simulink model "model_cnn"  (R2020a)
settings: Solver=VariableStepAuto  StartTime=0.0  StopTime=1e6/fs  RelTol=1e-3
PreLoadFcn:
  | setup_imports;
  | %dense2_numerictype = fixdt(1,18,10);
  | %conv1_numerictype = fixdt(1,18,21);
InitFcn:
  | % Intermediate signal dimensions
  | input_dim = [1, 2, 128];
  | layer1_dim = hInterConvLayerDims([1,3,1,64],input_dim,1); % dims : [C,H,W]
  | layer2_dim = hInterConvLayerDims([2,3,64,16],layer1_dim,1);% dims : [C,H,W]
  | layer3_dim = [1,128];
  | 
  | % Conv Layer 1 dimensions
  | conv1_dims = struct(...
  |     'input_dim',    input_dim,...       input_dim = C,H,W
  |     'filter_dim',   [1, 3, 1, 64],...  filter_dim = K,J,C,N
  |     'stride',       1,...
  |     'row_output',   3,...
  |     'output_dim',   layer1_dim);
  | 
  | % Conv Layer 2 dimensions
  | conv2_dims = struct(...
  |     'input_dim',    layer1_dim,...      input = C,H.W
  |     'filter_dim',   [2, 3, 64, 16],...  filter_dim = K,J,C,N
  |     'stride',       1,...
  |     'row_output',   2*3*64,...
  |     'output_dim',   layer2_dim);
  | 
  | % Dense Layer 1 dimensions
  | dense1_dims = struct(...
  |     'input_dim',    layer2_dim,...      input = C,H,W
  |     'weight_dim',   [1984, 128],...     weight_dim = H,W
  |     'output_dim',   layer3_dim);
  | 
  | % Load saved weights and input
  | setup_imports;
  | 
  | fs = 128e6;
  | fs_axi = 100e6;
  | R = 32;
values from neighbouring files (symbols this model uses):
  datatypeInput = X_test.numerictype    [setup_imports.m]
  gemm_wconv1 = fi(hInterleaveFilters(Wconv1),1,16)    [setup_imports.m]
  gemm_wconv2 = fi(hInterleaveFilters(Wconv2),1,16)    [setup_imports.m]
  wdense1 = fi(Wdense1,1,16)    [setup_imports.m]
  wdense2 = fi(Wdense2,1,16)    [setup_imports.m]
undefined symbols (not defined in the file or in its folder): ltehdlRAMinitPO2
libraries: hdlsllib x1022, dspsigops x3, dspsrcs4 x2
(part 5 of 23)

== system model_cnn/HDL CNN Model/Conv Layer 1/Layer 1 Mat-Vec Multiplier/adder54 ==
  In1 : Inport
  In2 : Inport  Port=2
  In3 : Inport  Port=3
  Data Type Conversion : DataTypeConversion  OutDataTypeStr=conv1_numerictype
  Multiply-Accumulate : hdlsllib/HDL Operations/Multiply-Accumulate  opMode=Streaming - using Number of Samples  initValueSetting=Dialog  initValue=0  initValueSetting2=Dialog  initValue2=0  initValueSetting3=Dialog  initValue3=0  num_samples=3  RndMeth2=Floor  RndMeth3=Floor  datatype2=Inherit: Inherit via back propagation  datatype3=accumoutdatatype1  validOut=on  endInandOut=on  startOut=on  countOut=on  dim=-1  DoSatur=off  parallel=off
      settings: SourceProductBaseCode=SL
  Terminator : Terminator
  Terminator1 : Terminator
  Terminator2 : Terminator
  dataOut : Outport
  wires:
  Data Type Conversion/1 -> dataOut/1
  ? -> Terminator1/1  "validOut"
  In2/1 -> Multiply-Accumulate/1
  In3/1 -> ?
  Multiply-Accumulate/1 -> Data Type Conversion/1
  ? -> Terminator/1  "countOut"
  In1/1 -> Multiply-Accumulate/2
  ? -> Terminator2/1  "vectorOutValid"

== system model_cnn/HDL CNN Model/Conv Layer 1/Layer 1 Mat-Vec Multiplier/adder55 ==
  In1 : Inport
  In2 : Inport  Port=2
  In3 : Inport  Port=3
  Data Type Conversion : DataTypeConversion  OutDataTypeStr=conv1_numerictype
  Multiply-Accumulate : hdlsllib/HDL Operations/Multiply-Accumulate  opMode=Streaming - using Number of Samples  initValueSetting=Dialog  initValue=0  initValueSetting2=Dialog  initValue2=0  initValueSetting3=Dialog  initValue3=0  num_samples=3  RndMeth2=Floor  RndMeth3=Floor  datatype2=Inherit: Inherit via back propagation  datatype3=accumoutdatatype1  validOut=on  endInandOut=on  startOut=on  countOut=on  dim=-1  DoSatur=off  parallel=off
      settings: SourceProductBaseCode=SL
  Terminator : Terminator
  Terminator1 : Terminator
  Terminator2 : Terminator
  dataOut : Outport
  wires:
  Data Type Conversion/1 -> dataOut/1
  ? -> Terminator1/1  "validOut"
  In2/1 -> Multiply-Accumulate/1
  In3/1 -> ?
  Multiply-Accumulate/1 -> Data Type Conversion/1
  ? -> Terminator/1  "countOut"
  In1/1 -> Multiply-Accumulate/2
  ? -> Terminator2/1  "vectorOutValid"

== system model_cnn/HDL CNN Model/Conv Layer 1/Layer 1 Mat-Vec Multiplier/adder56 ==
  In1 : Inport
  In2 : Inport  Port=2
  In3 : Inport  Port=3
  Data Type Conversion : DataTypeConversion  OutDataTypeStr=conv1_numerictype
  Multiply-Accumulate : hdlsllib/HDL Operations/Multiply-Accumulate  opMode=Streaming - using Number of Samples  initValueSetting=Dialog  initValue=0  initValueSetting2=Dialog  initValue2=0  initValueSetting3=Dialog  initValue3=0  num_samples=3  RndMeth2=Floor  RndMeth3=Floor  datatype2=Inherit: Inherit via back propagation  datatype3=accumoutdatatype1  validOut=on  endInandOut=on  startOut=on  countOut=on  dim=-1  DoSatur=off  parallel=off
      settings: SourceProductBaseCode=SL
  Terminator : Terminator
  Terminator1 : Terminator
  Terminator2 : Terminator
  dataOut : Outport
  wires:
  Data Type Conversion/1 -> dataOut/1
  ? -> Terminator1/1  "validOut"
  In2/1 -> Multiply-Accumulate/1
  In3/1 -> ?
  Multiply-Accumulate/1 -> Data Type Conversion/1
  ? -> Terminator/1  "countOut"
  In1/1 -> Multiply-Accumulate/2
  ? -> Terminator2/1  "vectorOutValid"

== system model_cnn/HDL CNN Model/Conv Layer 1/Layer 1 Mat-Vec Multiplier/adder57 ==
  In1 : Inport
  In2 : Inport  Port=2
  In3 : Inport  Port=3
  Data Type Conversion : DataTypeConversion  OutDataTypeStr=conv1_numerictype
  Multiply-Accumulate : hdlsllib/HDL Operations/Multiply-Accumulate  opMode=Streaming - using Number of Samples  initValueSetting=Dialog  initValue=0  initValueSetting2=Dialog  initValue2=0  initValueSetting3=Dialog  initValue3=0  num_samples=3  RndMeth2=Floor  RndMeth3=Floor  datatype2=Inherit: Inherit via back propagation  datatype3=accumoutdatatype1  validOut=on  endInandOut=on  startOut=on  countOut=on  dim=-1  DoSatur=off  parallel=off
      settings: SourceProductBaseCode=SL
  Terminator : Terminator
  Terminator1 : Terminator
  Terminator2 : Terminator
  dataOut : Outport
  wires:
  Data Type Conversion/1 -> dataOut/1
  ? -> Terminator1/1  "validOut"
  In2/1 -> Multiply-Accumulate/1
  In3/1 -> ?
  Multiply-Accumulate/1 -> Data Type Conversion/1
  ? -> Terminator/1  "countOut"
  In1/1 -> Multiply-Accumulate/2
  ? -> Terminator2/1  "vectorOutValid"

== system model_cnn/HDL CNN Model/Conv Layer 1/Layer 1 Mat-Vec Multiplier/adder58 ==
  In1 : Inport
  In2 : Inport  Port=2
  In3 : Inport  Port=3
  Data Type Conversion : DataTypeConversion  OutDataTypeStr=conv1_numerictype
  Multiply-Accumulate : hdlsllib/HDL Operations/Multiply-Accumulate  opMode=Streaming - using Number of Samples  initValueSetting=Dialog  initValue=0  initValueSetting2=Dialog  initValue2=0  initValueSetting3=Dialog  initValue3=0  num_samples=3  RndMeth2=Floor  RndMeth3=Floor  datatype2=Inherit: Inherit via back propagation  datatype3=accumoutdatatype1  validOut=on  endInandOut=on  startOut=on  countOut=on  dim=-1  DoSatur=off  parallel=off
      settings: SourceProductBaseCode=SL
  Terminator : Terminator
  Terminator1 : Terminator
  Terminator2 : Terminator
  dataOut : Outport
  wires:
  Data Type Conversion/1 -> dataOut/1
  ? -> Terminator1/1  "validOut"
  In2/1 -> Multiply-Accumulate/1
  In3/1 -> ?
  Multiply-Accumulate/1 -> Data Type Conversion/1
  ? -> Terminator/1  "countOut"
  In1/1 -> Multiply-Accumulate/2
  ? -> Terminator2/1  "vectorOutValid"

== system model_cnn/HDL CNN Model/Conv Layer 1/Layer 1 Mat-Vec Multiplier/adder59 ==
  In1 : Inport
  In2 : Inport  Port=2
  In3 : Inport  Port=3
  Data Type Conversion : DataTypeConversion  OutDataTypeStr=conv1_numerictype
  Multiply-Accumulate : hdlsllib/HDL Operations/Multiply-Accumulate  opMode=Streaming - using Number of Samples  initValueSetting=Dialog  initValue=0  initValueSetting2=Dialog  initValue2=0  initValueSetting3=Dialog  initValue3=0  num_samples=3  RndMeth2=Floor  RndMeth3=Floor  datatype2=Inherit: Inherit via back propagation  datatype3=accumoutdatatype1  validOut=on  endInandOut=on  startOut=on  countOut=on  dim=-1  DoSatur=off  parallel=off
      settings: SourceProductBaseCode=SL
  Terminator : Terminator
  Terminator1 : Terminator
  Terminator2 : Terminator
  dataOut : Outport
  wires:
  Data Type Conversion/1 -> dataOut/1
  ? -> Terminator1/1  "validOut"
  In2/1 -> Multiply-Accumulate/1
  In3/1 -> ?
  Multiply-Accumulate/1 -> Data Type Conversion/1
  ? -> Terminator/1  "countOut"
  In1/1 -> Multiply-Accumulate/2
  ? -> Terminator2/1  "vectorOutValid"

== system model_cnn/HDL CNN Model/Conv Layer 1/Layer 1 Mat-Vec Multiplier/adder6 ==
  In1 : Inport
  In2 : Inport  Port=2
  In3 : Inport  Port=3
  Data Type Conversion : DataTypeConversion  OutDataTypeStr=conv1_numerictype
  Multiply-Accumulate : hdlsllib/HDL Operations/Multiply-Accumulate  opMode=Streaming - using Number of Samples  initValueSetting=Dialog  initValue=0  initValueSetting2=Dialog  initValue2=0  initValueSetting3=Dialog  initValue3=0  num_samples=3  RndMeth2=Floor  RndMeth3=Floor  datatype2=Inherit: Inherit via back propagation  datatype3=accumoutdatatype1  validOut=on  endInandOut=on  startOut=on  countOut=on  dim=-1  DoSatur=off  parallel=off
      settings: SourceProductBaseCode=SL
  Terminator : Terminator
  Terminator1 : Terminator
  Terminator2 : Terminator
  dataOut : Outport
  wires:
  Data Type Conversion/1 -> dataOut/1
  ? -> Terminator1/1  "validOut"
  In2/1 -> Multiply-Accumulate/1
  In3/1 -> ?
  Multiply-Accumulate/1 -> Data Type Conversion/1
  ? -> Terminator/1  "countOut"
  In1/1 -> Multiply-Accumulate/2
  ? -> Terminator2/1  "vectorOutValid"

== system model_cnn/HDL CNN Model/Conv Layer 1/Layer 1 Mat-Vec Multiplier/adder60 ==
  In1 : Inport
  In2 : Inport  Port=2
  In3 : Inport  Port=3
  Data Type Conversion : DataTypeConversion  OutDataTypeStr=conv1_numerictype
  Multiply-Accumulate : hdlsllib/HDL Operations/Multiply-Accumulate  opMode=Streaming - using Number of Samples  initValueSetting=Dialog  initValue=0  initValueSetting2=Dialog  initValue2=0  initValueSetting3=Dialog  initValue3=0  num_samples=3  RndMeth2=Floor  RndMeth3=Floor  datatype2=Inherit: Inherit via back propagation  datatype3=accumoutdatatype1  validOut=on  endInandOut=on  startOut=on  countOut=on  dim=-1  DoSatur=off  parallel=off
      settings: SourceProductBaseCode=SL
  Terminator : Terminator
  Terminator1 : Terminator
  Terminator2 : Terminator
  dataOut : Outport
  wires:
  Data Type Conversion/1 -> dataOut/1
  ? -> Terminator1/1  "validOut"
  In2/1 -> Multiply-Accumulate/1
  In3/1 -> ?
  Multiply-Accumulate/1 -> Data Type Conversion/1
  ? -> Terminator/1  "countOut"
  In1/1 -> Multiply-Accumulate/2
  ? -> Terminator2/1  "vectorOutValid"

== system model_cnn/HDL CNN Model/Conv Layer 1/Layer 1 Mat-Vec Multiplier/adder61 ==
  In1 : Inport
  In2 : Inport  Port=2
  In3 : Inport  Port=3
  Data Type Conversion : DataTypeConversion  OutDataTypeStr=conv1_numerictype
  Multiply-Accumulate : hdlsllib/HDL Operations/Multiply-Accumulate  opMode=Streaming - using Number of Samples  initValueSetting=Dialog  initValue=0  initValueSetting2=Dialog  initValue2=0  initValueSetting3=Dialog  initValue3=0  num_samples=3  RndMeth2=Floor  RndMeth3=Floor  datatype2=Inherit: Inherit via back propagation  datatype3=accumoutdatatype1  validOut=on  endInandOut=on  startOut=on  countOut=on  dim=-1  DoSatur=off  parallel=off
      settings: SourceProductBaseCode=SL
  Terminator : Terminator
  Terminator1 : Terminator
  Terminator2 : Terminator
  dataOut : Outport
  wires:
  Data Type Conversion/1 -> dataOut/1
  ? -> Terminator1/1  "validOut"
  In2/1 -> Multiply-Accumulate/1
  In3/1 -> ?
  Multiply-Accumulate/1 -> Data Type Conversion/1
  ? -> Terminator/1  "countOut"
  In1/1 -> Multiply-Accumulate/2
  ? -> Terminator2/1  "vectorOutValid"

== system model_cnn/HDL CNN Model/Conv Layer 1/Layer 1 Mat-Vec Multiplier/adder62 ==
  In1 : Inport
  In2 : Inport  Port=2
  In3 : Inport  Port=3
  Data Type Conversion : DataTypeConversion  OutDataTypeStr=conv1_numerictype
  Multiply-Accumulate : hdlsllib/HDL Operations/Multiply-Accumulate  opMode=Streaming - using Number of Samples  initValueSetting=Dialog  initValue=0  initValueSetting2=Dialog  initValue2=0  initValueSetting3=Dialog  initValue3=0  num_samples=3  RndMeth2=Floor  RndMeth3=Floor  datatype2=Inherit: Inherit via back propagation  datatype3=accumoutdatatype1  validOut=on  endInandOut=on  startOut=on  countOut=on  dim=-1  DoSatur=off  parallel=off
      settings: SourceProductBaseCode=SL
  Terminator : Terminator
  Terminator1 : Terminator
  Terminator2 : Terminator
  dataOut : Outport
  wires:
  Data Type Conversion/1 -> dataOut/1
  ? -> Terminator1/1  "validOut"
  In2/1 -> Multiply-Accumulate/1
  In3/1 -> ?
  Multiply-Accumulate/1 -> Data Type Conversion/1
  ? -> Terminator/1  "countOut"
  In1/1 -> Multiply-Accumulate/2
  ? -> Terminator2/1  "vectorOutValid"

== system model_cnn/HDL CNN Model/Conv Layer 1/Layer 1 Mat-Vec Multiplier/adder63 ==
  In1 : Inport
  In2 : Inport  Port=2
  In3 : Inport  Port=3
  Data Type Conversion : DataTypeConversion  OutDataTypeStr=conv1_numerictype
  Multiply-Accumulate : hdlsllib/HDL Operations/Multiply-Accumulate  opMode=Streaming - using Number of Samples  initValueSetting=Dialog  initValue=0  initValueSetting2=Dialog  initValue2=0  initValueSetting3=Dialog  initValue3=0  num_samples=3  RndMeth2=Floor  RndMeth3=Floor  datatype2=Inherit: Inherit via back propagation  datatype3=accumoutdatatype1  validOut=on  endInandOut=on  startOut=on  countOut=on  dim=-1  DoSatur=off  parallel=off
      settings: SourceProductBaseCode=SL
  Terminator : Terminator
  Terminator1 : Terminator
  Terminator2 : Terminator
  dataOut : Outport
  wires:
  Data Type Conversion/1 -> dataOut/1
  ? -> Terminator1/1  "validOut"
  In2/1 -> Multiply-Accumulate/1
  In3/1 -> ?
  Multiply-Accumulate/1 -> Data Type Conversion/1
  ? -> Terminator/1  "countOut"
  In1/1 -> Multiply-Accumulate/2
  ? -> Terminator2/1  "vectorOutValid"

== system model_cnn/HDL CNN Model/Conv Layer 1/Layer 1 Mat-Vec Multiplier/adder7 ==
  In1 : Inport
  In2 : Inport  Port=2
  In3 : Inport  Port=3
  Data Type Conversion : DataTypeConversion  OutDataTypeStr=conv1_numerictype
  Multiply-Accumulate : hdlsllib/HDL Operations/Multiply-Accumulate  opMode=Streaming - using Number of Samples  initValueSetting=Dialog  initValue=0  initValueSetting2=Dialog  initValue2=0  initValueSetting3=Dialog  initValue3=0  num_samples=3  RndMeth2=Floor  RndMeth3=Floor  datatype2=Inherit: Inherit via back propagation  datatype3=accumoutdatatype1  validOut=on  endInandOut=on  startOut=on  countOut=on  dim=-1  DoSatur=off  parallel=off
      settings: SourceProductBaseCode=SL
  Terminator : Terminator
  Terminator1 : Terminator
  Terminator2 : Terminator
  dataOut : Outport
  wires:
  Data Type Conversion/1 -> dataOut/1
  ? -> Terminator1/1  "validOut"
  In2/1 -> Multiply-Accumulate/1
  In3/1 -> ?
  Multiply-Accumulate/1 -> Data Type Conversion/1
  ? -> Terminator/1  "countOut"
  In1/1 -> Multiply-Accumulate/2
  ? -> Terminator2/1  "vectorOutValid"

== system model_cnn/HDL CNN Model/Conv Layer 1/Layer 1 Mat-Vec Multiplier/adder8 ==
  In1 : Inport
  In2 : Inport  Port=2
  In3 : Inport  Port=3
  Data Type Conversion : DataTypeConversion  OutDataTypeStr=conv1_numerictype
  Multiply-Accumulate : hdlsllib/HDL Operations/Multiply-Accumulate  opMode=Streaming - using Number of Samples  initValueSetting=Dialog  initValue=0  initValueSetting2=Dialog  initValue2=0  initValueSetting3=Dialog  initValue3=0  num_samples=3  RndMeth2=Floor  RndMeth3=Floor  datatype2=Inherit: Inherit via back propagation  datatype3=accumoutdatatype1  validOut=on  endInandOut=on  startOut=on  countOut=on  dim=-1  DoSatur=off  parallel=off
      settings: SourceProductBaseCode=SL
  Terminator : Terminator
  Terminator1 : Terminator
  Terminator2 : Terminator
  dataOut : Outport
  wires:
  Data Type Conversion/1 -> dataOut/1
  ? -> Terminator1/1  "validOut"
  In2/1 -> Multiply-Accumulate/1
  In3/1 -> ?
  Multiply-Accumulate/1 -> Data Type Conversion/1
  ? -> Terminator/1  "countOut"
  In1/1 -> Multiply-Accumulate/2
  ? -> Terminator2/1  "vectorOutValid"

== system model_cnn/HDL CNN Model/Conv Layer 1/Layer 1 Mat-Vec Multiplier/adder9 ==
  In1 : Inport
  In2 : Inport  Port=2
  In3 : Inport  Port=3
  Data Type Conversion : DataTypeConversion  OutDataTypeStr=conv1_numerictype
  Multiply-Accumulate : hdlsllib/HDL Operations/Multiply-Accumulate  opMode=Streaming - using Number of Samples  initValueSetting=Dialog  initValue=0  initValueSetting2=Dialog  initValue2=0  initValueSetting3=Dialog  initValue3=0  num_samples=3  RndMeth2=Floor  RndMeth3=Floor  datatype2=Inherit: Inherit via back propagation  datatype3=accumoutdatatype1  validOut=on  endInandOut=on  startOut=on  countOut=on  dim=-1  DoSatur=off  parallel=off
      settings: SourceProductBaseCode=SL
  Terminator : Terminator
  Terminator1 : Terminator
  Terminator2 : Terminator
  dataOut : Outport
  wires:
  Data Type Conversion/1 -> dataOut/1
  ? -> Terminator1/1  "validOut"
  In2/1 -> Multiply-Accumulate/1
  In3/1 -> ?
  Multiply-Accumulate/1 -> Data Type Conversion/1
  ? -> Terminator/1  "countOut"
  In1/1 -> Multiply-Accumulate/2
  ? -> Terminator2/1  "vectorOutValid"

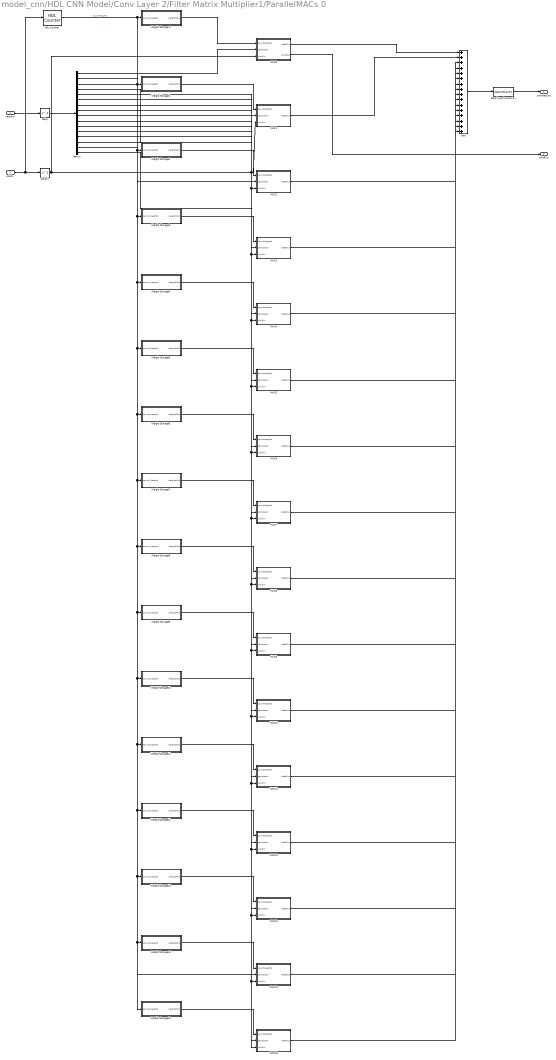
== system model_cnn/HDL CNN Model/Conv Layer 2/Filter Matrix Multiplier1/ParallelMACs 0 ==
  vectorIn : Inport
  validIn : Inport  Port=2
  Add : Sum  Inputs=++++++++++++++++  AccumDataTypeStr=accumoutdatatype2  OutDataTypeStr=accumoutdatatype2
  Data Type Conversion : DataTypeConversion  OutDataTypeStr=datatypeLayer2
  Delay : Delay  DelayLength=1
  Delay1 : Delay  DelayLength=1
  Demux : Demux  Outputs=16
  HDL Counter : hdlsllib/Sources/HDL Counter  CountType=Count limited  CountInit=0  CountStep=1  CountMax=24-1  CountFromType=Initial value  CountFrom=0  CountResetPort=off  CountLoadPort=off  CountEnbPort=on  CountDirPort=off  CountDataType=Unsigned  CountWordLen=ceil(log2(24))  CountFracLen=0  CountSampTime=1
  MAC0 : Subsystem
  MAC1 : Subsystem
  MAC10 : Subsystem
  MAC11 : Subsystem
  MAC12 : Subsystem
  MAC13 : Subsystem
  MAC14 : Subsystem
  MAC15 : Subsystem
  MAC2 : Subsystem
  MAC3 : Subsystem
  MAC4 : Subsystem
  MAC5 : Subsystem
  MAC6 : Subsystem
  MAC7 : Subsystem
  MAC8 : Subsystem
  MAC9 : Subsystem
  Weight Storage 0 : Subsystem  mask{dim=filter_dim, dim2=1}
      mask prompts: dim "Filter Selection"; dim2 "Slice Selection"
  Weight Storage1 : Subsystem  mask{dim=filter_dim, dim2=2}
      mask prompts: dim "Filter Selection"; dim2 "Slice Selection"
  Weight Storage10 : Subsystem  mask{dim=filter_dim, dim2=11}
      mask prompts: dim "Filter Selection"; dim2 "Slice Selection"
  Weight Storage11 : Subsystem  mask{dim=filter_dim, dim2=12}
      mask prompts: dim "Filter Selection"; dim2 "Slice Selection"
  Weight Storage12 : Subsystem  mask{dim=filter_dim, dim2=13}
      mask prompts: dim "Filter Selection"; dim2 "Slice Selection"
  Weight Storage13 : Subsystem  mask{dim=filter_dim, dim2=14}
      mask prompts: dim "Filter Selection"; dim2 "Slice Selection"
  Weight Storage14 : Subsystem  mask{dim=filter_dim, dim2=15}
      mask prompts: dim "Filter Selection"; dim2 "Slice Selection"
  Weight Storage15 : Subsystem  mask{dim=filter_dim, dim2=16}
      mask prompts: dim "Filter Selection"; dim2 "Slice Selection"
  Weight Storage2 : Subsystem  mask{dim=filter_dim, dim2=3}
      mask prompts: dim "Filter Selection"; dim2 "Slice Selection"
  Weight Storage3 : Subsystem  mask{dim=filter_dim, dim2=4}
      mask prompts: dim "Filter Selection"; dim2 "Slice Selection"
  Weight Storage4 : Subsystem  mask{dim=filter_dim, dim2=5}
      mask prompts: dim "Filter Selection"; dim2 "Slice Selection"
  Weight Storage5 : Subsystem  mask{dim=filter_dim, dim2=6}
      mask prompts: dim "Filter Selection"; dim2 "Slice Selection"
  Weight Storage6 : Subsystem  mask{dim=filter_dim, dim2=7}
      mask prompts: dim "Filter Selection"; dim2 "Slice Selection"
  Weight Storage7 : Subsystem  mask{dim=filter_dim, dim2=8}
      mask prompts: dim "Filter Selection"; dim2 "Slice Selection"
  Weight Storage8 : Subsystem  mask{dim=filter_dim, dim2=9}
      mask prompts: dim "Filter Selection"; dim2 "Slice Selection"
  Weight Storage9 : Subsystem  mask{dim=filter_dim, dim2=10}
      mask prompts: dim "Filter Selection"; dim2 "Slice Selection"
  samplesOut : Outport
  validOut : Outport  Port=2
  wires:
  MAC0/2(validOut) -> validOut/1
  Demux/16 -> MAC15/2(samplesIn)
  MAC15/1(dataOut) -> Add/16
  Weight Storage15/1(weightsOut) -> MAC15/1(countWeights)
  Demux/15 -> MAC14/2(samplesIn)
  MAC14/1(dataOut) -> Add/15
  Weight Storage14/1(weightsOut) -> MAC14/1(countWeights)
  Demux/14 -> MAC13/2(samplesIn)
  MAC13/1(dataOut) -> Add/14
  Weight Storage13/1(weightsOut) -> MAC13/1(countWeights)
  Demux/13 -> MAC12/2(samplesIn)
  MAC12/1(dataOut) -> Add/13
  Weight Storage12/1(weightsOut) -> MAC12/1(countWeights)
  Demux/12 -> MAC11/2(samplesIn)
  MAC11/1(dataOut) -> Add/12
  Weight Storage11/1(weightsOut) -> MAC11/1(countWeights)
  Demux/11 -> MAC10/2(samplesIn)
  MAC10/1(dataOut) -> Add/11
  Weight Storage10/1(weightsOut) -> MAC10/1(countWeights)
  Demux/10 -> MAC9/2(samplesIn)
  MAC9/1(dataOut) -> Add/10
  Weight Storage9/1(weightsOut) -> MAC9/1(countWeights)
  Demux/9 -> MAC8/2(samplesIn)
  MAC8/1(dataOut) -> Add/9
  Weight Storage8/1(weightsOut) -> MAC8/1(countWeights)
  Demux/8 -> MAC7/2(samplesIn)
  MAC7/1(dataOut) -> Add/8
  Weight Storage7/1(weightsOut) -> MAC7/1(countWeights)
  Demux/7 -> MAC6/2(samplesIn)
  MAC6/1(dataOut) -> Add/7
  Weight Storage6/1(weightsOut) -> MAC6/1(countWeights)
  Demux/6 -> MAC5/2(samplesIn)
  MAC5/1(dataOut) -> Add/6
  Weight Storage5/1(weightsOut) -> MAC5/1(countWeights)
  Demux/5 -> MAC4/2(samplesIn)
  MAC4/1(dataOut) -> Add/5
  Weight Storage4/1(weightsOut) -> MAC4/1(countWeights)
  Demux/4 -> MAC3/2(samplesIn)
  MAC3/1(dataOut) -> Add/4
  Weight Storage3/1(weightsOut) -> MAC3/1(countWeights)
  Demux/3 -> MAC2/2(samplesIn)
  MAC2/1(dataOut) -> Add/3
  Weight Storage2/1(weightsOut) -> MAC2/1(countWeights)
  Demux/2 -> MAC1/2(samplesIn)
  MAC1/1(dataOut) -> Add/2
  Weight Storage1/1(weightsOut) -> MAC1/1(countWeights)
  Add/1 -> Data Type Conversion/1
  Weight Storage 0/1(weightsOut) -> MAC0/1(countWeights)
  validIn/1 -> HDL Counter/1, Delay1/1
  HDL Counter/1 -> Weight Storage15/1(count_Weights), Weight Storage14/1(count_Weights), Weight Storage13/1(count_Weights), Weight Storage12/1(count_Weights), Weight Storage11/1(count_Weights), Weight Storage10/1(count_Weights), Weight Storage9/1(count_Weights), Weight Storage8/1(count_Weights), Weight Storage7/1(count_Weights), Weight Storage6/1(count_Weights), Weight Storage5/1(count_Weights), Weight Storage4/1(count_Weights), Weight Storage3/1(count_Weights), Weight Storage2/1(count_Weights), Weight Storage1/1(count_Weights), Weight Storage 0/1(count_Weights)  "countWeights"
  Delay/1 -> Demux/1
  vectorIn/1 -> Delay/1
  Delay1/1 -> MAC0/3(validIn), MAC1/3(validIn), MAC2/3(validIn), MAC3/3(validIn), MAC4/3(validIn), MAC5/3(validIn), MAC6/3(validIn), MAC7/3(validIn), MAC8/3(validIn), MAC9/3(validIn), MAC10/3(validIn), MAC11/3(validIn), MAC12/3(validIn), MAC13/3(validIn), MAC15/3(validIn), MAC14/3(validIn)
  MAC0/1(dataOut) -> Add/1
  Demux/1 -> MAC0/2(samplesIn)
  Data Type Conversion/1 -> samplesOut/1

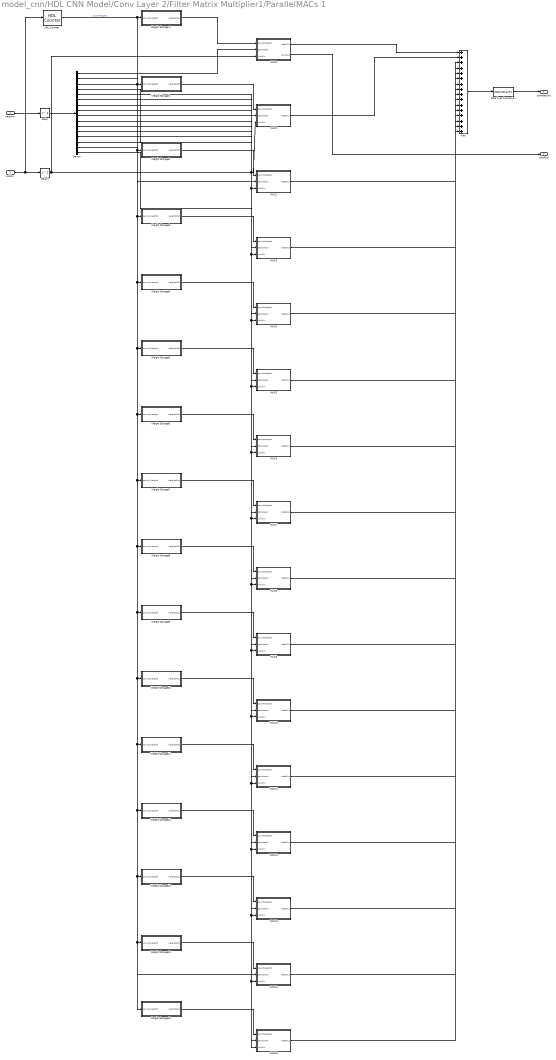
== system model_cnn/HDL CNN Model/Conv Layer 2/Filter Matrix Multiplier1/ParallelMACs 1 ==
  vectorIn : Inport
  validIn : Inport  Port=2
  Add : Sum  Inputs=++++++++++++++++  AccumDataTypeStr=accumoutdatatype2  OutDataTypeStr=accumoutdatatype2
  Data Type Conversion : DataTypeConversion  OutDataTypeStr=datatypeLayer2
  Delay : Delay  DelayLength=1
  Delay1 : Delay  DelayLength=1
  Demux : Demux  Outputs=16
  HDL Counter : hdlsllib/Sources/HDL Counter  CountType=Count limited  CountInit=0  CountStep=1  CountMax=24-1  CountFromType=Initial value  CountFrom=0  CountResetPort=off  CountLoadPort=off  CountEnbPort=on  CountDirPort=off  CountDataType=Unsigned  CountWordLen=ceil(log2(24))  CountFracLen=0  CountSampTime=1
  MAC0 : Subsystem
  MAC1 : Subsystem
  MAC10 : Subsystem
  MAC11 : Subsystem
  MAC12 : Subsystem
  MAC13 : Subsystem
  MAC14 : Subsystem
  MAC15 : Subsystem
  MAC2 : Subsystem
  MAC3 : Subsystem
  MAC4 : Subsystem
  MAC5 : Subsystem
  MAC6 : Subsystem
  MAC7 : Subsystem
  MAC8 : Subsystem
  MAC9 : Subsystem
  Weight Storage 0 : Subsystem  mask{dim=filter_dim, dim2=1}
      mask prompts: dim "Filter Selection"; dim2 "Slice Selection"
  Weight Storage1 : Subsystem  mask{dim=filter_dim, dim2=2}
      mask prompts: dim "Filter Selection"; dim2 "Slice Selection"
  Weight Storage10 : Subsystem  mask{dim=filter_dim, dim2=11}
      mask prompts: dim "Filter Selection"; dim2 "Slice Selection"
  Weight Storage11 : Subsystem  mask{dim=filter_dim, dim2=12}
      mask prompts: dim "Filter Selection"; dim2 "Slice Selection"
  Weight Storage12 : Subsystem  mask{dim=filter_dim, dim2=13}
      mask prompts: dim "Filter Selection"; dim2 "Slice Selection"
  Weight Storage13 : Subsystem  mask{dim=filter_dim, dim2=14}
      mask prompts: dim "Filter Selection"; dim2 "Slice Selection"
  Weight Storage14 : Subsystem  mask{dim=filter_dim, dim2=15}
      mask prompts: dim "Filter Selection"; dim2 "Slice Selection"
  Weight Storage15 : Subsystem  mask{dim=filter_dim, dim2=16}
      mask prompts: dim "Filter Selection"; dim2 "Slice Selection"
  Weight Storage2 : Subsystem  mask{dim=filter_dim, dim2=3}
      mask prompts: dim "Filter Selection"; dim2 "Slice Selection"
  Weight Storage3 : Subsystem  mask{dim=filter_dim, dim2=4}
      mask prompts: dim "Filter Selection"; dim2 "Slice Selection"
  Weight Storage4 : Subsystem  mask{dim=filter_dim, dim2=5}
      mask prompts: dim "Filter Selection"; dim2 "Slice Selection"
  Weight Storage5 : Subsystem  mask{dim=filter_dim, dim2=6}
      mask prompts: dim "Filter Selection"; dim2 "Slice Selection"
  Weight Storage6 : Subsystem  mask{dim=filter_dim, dim2=7}
      mask prompts: dim "Filter Selection"; dim2 "Slice Selection"
  Weight Storage7 : Subsystem  mask{dim=filter_dim, dim2=8}
      mask prompts: dim "Filter Selection"; dim2 "Slice Selection"
  Weight Storage8 : Subsystem  mask{dim=filter_dim, dim2=9}
      mask prompts: dim "Filter Selection"; dim2 "Slice Selection"
  Weight Storage9 : Subsystem  mask{dim=filter_dim, dim2=10}
      mask prompts: dim "Filter Selection"; dim2 "Slice Selection"
  samplesOut : Outport
  validOut : Outport  Port=2
  wires:
  Data Type Conversion/1 -> samplesOut/1
  Demux/1 -> MAC0/2(samplesIn)
  MAC0/1(dataOut) -> Add/1
  Delay1/1 -> MAC14/3(validIn), MAC15/3(validIn), MAC13/3(validIn), MAC12/3(validIn), MAC11/3(validIn), MAC10/3(validIn), MAC9/3(validIn), MAC8/3(validIn), MAC7/3(validIn), MAC6/3(validIn), MAC5/3(validIn), MAC4/3(validIn), MAC3/3(validIn), MAC2/3(validIn), MAC1/3(validIn), MAC0/3(validIn)
  vectorIn/1 -> Delay/1
  Delay/1 -> Demux/1
  HDL Counter/1 -> Weight Storage 0/1(count_Weights), Weight Storage1/1(count_Weights), Weight Storage2/1(count_Weights), Weight Storage3/1(count_Weights), Weight Storage4/1(count_Weights), Weight Storage5/1(count_Weights), Weight Storage6/1(count_Weights), Weight Storage7/1(count_Weights), Weight Storage8/1(count_Weights), Weight Storage9/1(count_Weights), Weight Storage10/1(count_Weights), Weight Storage11/1(count_Weights), Weight Storage12/1(count_Weights), Weight Storage13/1(count_Weights), Weight Storage14/1(count_Weights), Weight Storage15/1(count_Weights)  "countWeights"
  validIn/1 -> Delay1/1, HDL Counter/1
  Weight Storage 0/1(weightsOut) -> MAC0/1(countWeights)
  Add/1 -> Data Type Conversion/1
  Weight Storage1/1(weightsOut) -> MAC1/1(countWeights)
  MAC1/1(dataOut) -> Add/2
  Demux/2 -> MAC1/2(samplesIn)
  Weight Storage2/1(weightsOut) -> MAC2/1(countWeights)
  MAC2/1(dataOut) -> Add/3
  Demux/3 -> MAC2/2(samplesIn)
  Weight Storage3/1(weightsOut) -> MAC3/1(countWeights)
  MAC3/1(dataOut) -> Add/4
  Demux/4 -> MAC3/2(samplesIn)
  Weight Storage4/1(weightsOut) -> MAC4/1(countWeights)
  MAC4/1(dataOut) -> Add/5
  Demux/5 -> MAC4/2(samplesIn)
  Weight Storage5/1(weightsOut) -> MAC5/1(countWeights)
  MAC5/1(dataOut) -> Add/6
  Demux/6 -> MAC5/2(samplesIn)
  Weight Storage6/1(weightsOut) -> MAC6/1(countWeights)
  MAC6/1(dataOut) -> Add/7
  Demux/7 -> MAC6/2(samplesIn)
  Weight Storage7/1(weightsOut) -> MAC7/1(countWeights)
  MAC7/1(dataOut) -> Add/8
  Demux/8 -> MAC7/2(samplesIn)
  Weight Storage8/1(weightsOut) -> MAC8/1(countWeights)
  MAC8/1(dataOut) -> Add/9
  Demux/9 -> MAC8/2(samplesIn)
  Weight Storage9/1(weightsOut) -> MAC9/1(countWeights)
  MAC9/1(dataOut) -> Add/10
  Demux/10 -> MAC9/2(samplesIn)
  Weight Storage10/1(weightsOut) -> MAC10/1(countWeights)
  MAC10/1(dataOut) -> Add/11
  Demux/11 -> MAC10/2(samplesIn)
  Weight Storage11/1(weightsOut) -> MAC11/1(countWeights)
  MAC11/1(dataOut) -> Add/12
  Demux/12 -> MAC11/2(samplesIn)
  Weight Storage12/1(weightsOut) -> MAC12/1(countWeights)
  MAC12/1(dataOut) -> Add/13
  Demux/13 -> MAC12/2(samplesIn)
  Weight Storage13/1(weightsOut) -> MAC13/1(countWeights)
  MAC13/1(dataOut) -> Add/14
  Demux/14 -> MAC13/2(samplesIn)
  Weight Storage14/1(weightsOut) -> MAC14/1(countWeights)
  MAC14/1(dataOut) -> Add/15
  Demux/15 -> MAC14/2(samplesIn)
  Weight Storage15/1(weightsOut) -> MAC15/1(countWeights)
  MAC15/1(dataOut) -> Add/16
  Demux/16 -> MAC15/2(samplesIn)
  MAC0/2(validOut) -> validOut/1

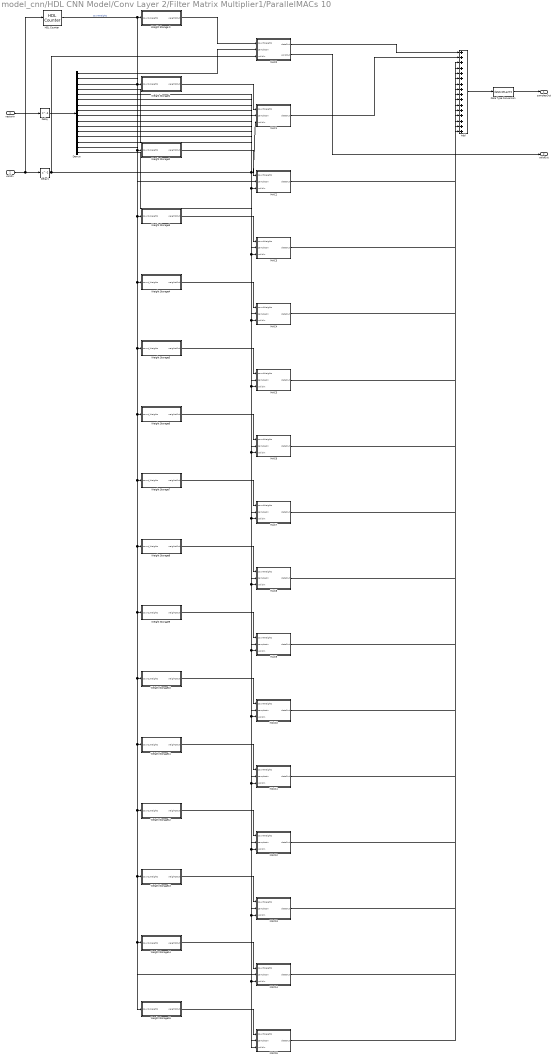
== system model_cnn/HDL CNN Model/Conv Layer 2/Filter Matrix Multiplier1/ParallelMACs 10 ==
  vectorIn : Inport
  validIn : Inport  Port=2
  Add : Sum  Inputs=++++++++++++++++  AccumDataTypeStr=accumoutdatatype2  OutDataTypeStr=accumoutdatatype2
  Data Type Conversion : DataTypeConversion  OutDataTypeStr=datatypeLayer2
  Delay : Delay  DelayLength=1
  Delay1 : Delay  DelayLength=1
  Demux : Demux  Outputs=16
  HDL Counter : hdlsllib/Sources/HDL Counter  CountType=Count limited  CountInit=0  CountStep=1  CountMax=24-1  CountFromType=Initial value  CountFrom=0  CountResetPort=off  CountLoadPort=off  CountEnbPort=on  CountDirPort=off  CountDataType=Unsigned  CountWordLen=ceil(log2(24))  CountFracLen=0  CountSampTime=1
  MAC0 : Subsystem
  MAC1 : Subsystem
  MAC10 : Subsystem
  MAC11 : Subsystem
  MAC12 : Subsystem
  MAC13 : Subsystem
  MAC14 : Subsystem
  MAC15 : Subsystem
  MAC2 : Subsystem
  MAC3 : Subsystem
  MAC4 : Subsystem
  MAC5 : Subsystem
  MAC6 : Subsystem
  MAC7 : Subsystem
  MAC8 : Subsystem
  MAC9 : Subsystem
  Weight Storage 0 : Subsystem  mask{dim=filter_dim, dim2=1}
      mask prompts: dim "Filter Selection"; dim2 "Slice Selection"
  Weight Storage1 : Subsystem  mask{dim=filter_dim, dim2=2}
      mask prompts: dim "Filter Selection"; dim2 "Slice Selection"
  Weight Storage10 : Subsystem  mask{dim=filter_dim, dim2=11}
      mask prompts: dim "Filter Selection"; dim2 "Slice Selection"
  Weight Storage11 : Subsystem  mask{dim=filter_dim, dim2=12}
      mask prompts: dim "Filter Selection"; dim2 "Slice Selection"
  Weight Storage12 : Subsystem  mask{dim=filter_dim, dim2=13}
      mask prompts: dim "Filter Selection"; dim2 "Slice Selection"
  Weight Storage13 : Subsystem  mask{dim=filter_dim, dim2=14}
      mask prompts: dim "Filter Selection"; dim2 "Slice Selection"
  Weight Storage14 : Subsystem  mask{dim=filter_dim, dim2=15}
      mask prompts: dim "Filter Selection"; dim2 "Slice Selection"
  Weight Storage15 : Subsystem  mask{dim=filter_dim, dim2=16}
      mask prompts: dim "Filter Selection"; dim2 "Slice Selection"
  Weight Storage2 : Subsystem  mask{dim=filter_dim, dim2=3}
      mask prompts: dim "Filter Selection"; dim2 "Slice Selection"
  Weight Storage3 : Subsystem  mask{dim=filter_dim, dim2=4}
      mask prompts: dim "Filter Selection"; dim2 "Slice Selection"
  Weight Storage4 : Subsystem  mask{dim=filter_dim, dim2=5}
      mask prompts: dim "Filter Selection"; dim2 "Slice Selection"
  Weight Storage5 : Subsystem  mask{dim=filter_dim, dim2=6}
      mask prompts: dim "Filter Selection"; dim2 "Slice Selection"
  Weight Storage6 : Subsystem  mask{dim=filter_dim, dim2=7}
      mask prompts: dim "Filter Selection"; dim2 "Slice Selection"
  Weight Storage7 : Subsystem  mask{dim=filter_dim, dim2=8}
      mask prompts: dim "Filter Selection"; dim2 "Slice Selection"
  Weight Storage8 : Subsystem  mask{dim=filter_dim, dim2=9}
      mask prompts: dim "Filter Selection"; dim2 "Slice Selection"
  Weight Storage9 : Subsystem  mask{dim=filter_dim, dim2=10}
      mask prompts: dim "Filter Selection"; dim2 "Slice Selection"
  samplesOut : Outport
  validOut : Outport  Port=2
  wires:
  MAC0/2(validOut) -> validOut/1
  Demux/16 -> MAC15/2(samplesIn)
  MAC15/1(dataOut) -> Add/16
  Weight Storage15/1(weightsOut) -> MAC15/1(countWeights)
  Demux/15 -> MAC14/2(samplesIn)
  MAC14/1(dataOut) -> Add/15
  Weight Storage14/1(weightsOut) -> MAC14/1(countWeights)
  Demux/14 -> MAC13/2(samplesIn)
  MAC13/1(dataOut) -> Add/14
  Weight Storage13/1(weightsOut) -> MAC13/1(countWeights)
  Demux/13 -> MAC12/2(samplesIn)
  MAC12/1(dataOut) -> Add/13
  Weight Storage12/1(weightsOut) -> MAC12/1(countWeights)
  Demux/12 -> MAC11/2(samplesIn)
  MAC11/1(dataOut) -> Add/12
  Weight Storage11/1(weightsOut) -> MAC11/1(countWeights)
  Demux/11 -> MAC10/2(samplesIn)
  MAC10/1(dataOut) -> Add/11
  Weight Storage10/1(weightsOut) -> MAC10/1(countWeights)
  Demux/10 -> MAC9/2(samplesIn)
  MAC9/1(dataOut) -> Add/10
  Weight Storage9/1(weightsOut) -> MAC9/1(countWeights)
  Demux/9 -> MAC8/2(samplesIn)
  MAC8/1(dataOut) -> Add/9
  Weight Storage8/1(weightsOut) -> MAC8/1(countWeights)
  Demux/8 -> MAC7/2(samplesIn)
  MAC7/1(dataOut) -> Add/8
  Weight Storage7/1(weightsOut) -> MAC7/1(countWeights)
  Demux/7 -> MAC6/2(samplesIn)
  MAC6/1(dataOut) -> Add/7
  Weight Storage6/1(weightsOut) -> MAC6/1(countWeights)
  Demux/6 -> MAC5/2(samplesIn)
  MAC5/1(dataOut) -> Add/6
  Weight Storage5/1(weightsOut) -> MAC5/1(countWeights)
  Demux/5 -> MAC4/2(samplesIn)
  MAC4/1(dataOut) -> Add/5
  Weight Storage4/1(weightsOut) -> MAC4/1(countWeights)
  Demux/4 -> MAC3/2(samplesIn)
  MAC3/1(dataOut) -> Add/4
  Weight Storage3/1(weightsOut) -> MAC3/1(countWeights)
  Demux/3 -> MAC2/2(samplesIn)
  MAC2/1(dataOut) -> Add/3
  Weight Storage2/1(weightsOut) -> MAC2/1(countWeights)
  Demux/2 -> MAC1/2(samplesIn)
  MAC1/1(dataOut) -> Add/2
  Weight Storage1/1(weightsOut) -> MAC1/1(countWeights)
  Add/1 -> Data Type Conversion/1
  Weight Storage 0/1(weightsOut) -> MAC0/1(countWeights)
  validIn/1 -> HDL Counter/1, Delay1/1
  HDL Counter/1 -> Weight Storage15/1(count_Weights), Weight Storage14/1(count_Weights), Weight Storage13/1(count_Weights), Weight Storage12/1(count_Weights), Weight Storage11/1(count_Weights), Weight Storage10/1(count_Weights), Weight Storage9/1(count_Weights), Weight Storage8/1(count_Weights), Weight Storage7/1(count_Weights), Weight Storage6/1(count_Weights), Weight Storage5/1(count_Weights), Weight Storage4/1(count_Weights), Weight Storage3/1(count_Weights), Weight Storage2/1(count_Weights), Weight Storage1/1(count_Weights), Weight Storage 0/1(count_Weights)  "countWeights"
  Delay/1 -> Demux/1
  vectorIn/1 -> Delay/1
  Delay1/1 -> MAC0/3(validIn), MAC1/3(validIn), MAC2/3(validIn), MAC3/3(validIn), MAC4/3(validIn), MAC5/3(validIn), MAC6/3(validIn), MAC7/3(validIn), MAC8/3(validIn), MAC9/3(validIn), MAC10/3(validIn), MAC11/3(validIn), MAC12/3(validIn), MAC13/3(validIn), MAC15/3(validIn), MAC14/3(validIn)
  MAC0/1(dataOut) -> Add/1
  Demux/1 -> MAC0/2(samplesIn)
  Data Type Conversion/1 -> samplesOut/1

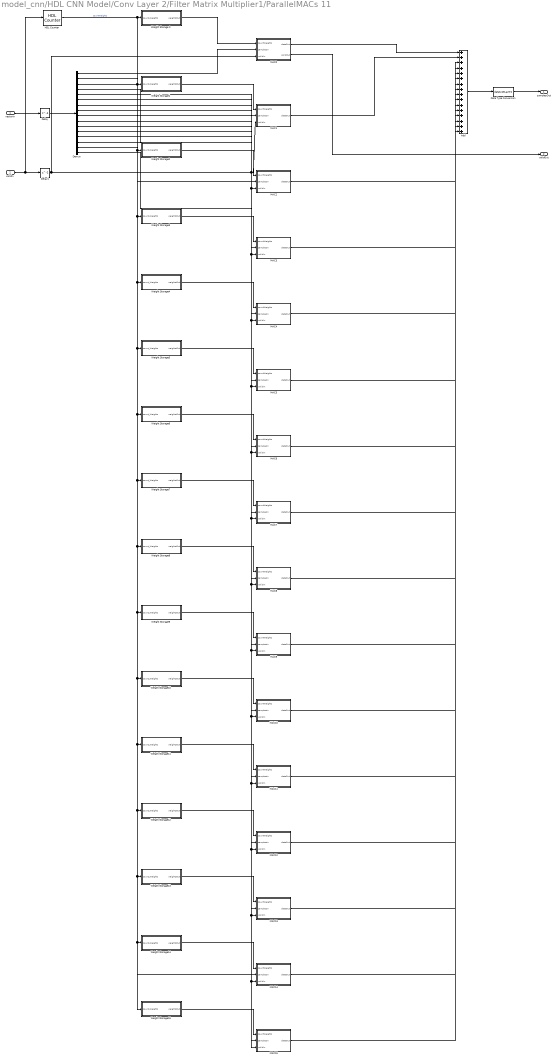
== system model_cnn/HDL CNN Model/Conv Layer 2/Filter Matrix Multiplier1/ParallelMACs 11 ==
  vectorIn : Inport
  validIn : Inport  Port=2
  Add : Sum  Inputs=++++++++++++++++  AccumDataTypeStr=accumoutdatatype2  OutDataTypeStr=accumoutdatatype2
  Data Type Conversion : DataTypeConversion  OutDataTypeStr=datatypeLayer2
  Delay : Delay  DelayLength=1
  Delay1 : Delay  DelayLength=1
  Demux : Demux  Outputs=16
  HDL Counter : hdlsllib/Sources/HDL Counter  CountType=Count limited  CountInit=0  CountStep=1  CountMax=24-1  CountFromType=Initial value  CountFrom=0  CountResetPort=off  CountLoadPort=off  CountEnbPort=on  CountDirPort=off  CountDataType=Unsigned  CountWordLen=ceil(log2(24))  CountFracLen=0  CountSampTime=1
  MAC0 : Subsystem
  MAC1 : Subsystem
  MAC10 : Subsystem
  MAC11 : Subsystem
  MAC12 : Subsystem
  MAC13 : Subsystem
  MAC14 : Subsystem
  MAC15 : Subsystem
  MAC2 : Subsystem
  MAC3 : Subsystem
  MAC4 : Subsystem
  MAC5 : Subsystem
  MAC6 : Subsystem
  MAC7 : Subsystem
  MAC8 : Subsystem
  MAC9 : Subsystem
  Weight Storage 0 : Subsystem  mask{dim=filter_dim, dim2=1}
      mask prompts: dim "Filter Selection"; dim2 "Slice Selection"
  Weight Storage1 : Subsystem  mask{dim=filter_dim, dim2=2}
      mask prompts: dim "Filter Selection"; dim2 "Slice Selection"
  Weight Storage10 : Subsystem  mask{dim=filter_dim, dim2=11}
      mask prompts: dim "Filter Selection"; dim2 "Slice Selection"
  Weight Storage11 : Subsystem  mask{dim=filter_dim, dim2=12}
      mask prompts: dim "Filter Selection"; dim2 "Slice Selection"
  Weight Storage12 : Subsystem  mask{dim=filter_dim, dim2=13}
      mask prompts: dim "Filter Selection"; dim2 "Slice Selection"
  Weight Storage13 : Subsystem  mask{dim=filter_dim, dim2=14}
      mask prompts: dim "Filter Selection"; dim2 "Slice Selection"
  Weight Storage14 : Subsystem  mask{dim=filter_dim, dim2=15}
      mask prompts: dim "Filter Selection"; dim2 "Slice Selection"
  Weight Storage15 : Subsystem  mask{dim=filter_dim, dim2=16}
      mask prompts: dim "Filter Selection"; dim2 "Slice Selection"
  Weight Storage2 : Subsystem  mask{dim=filter_dim, dim2=3}
      mask prompts: dim "Filter Selection"; dim2 "Slice Selection"
  Weight Storage3 : Subsystem  mask{dim=filter_dim, dim2=4}
      mask prompts: dim "Filter Selection"; dim2 "Slice Selection"
  Weight Storage4 : Subsystem  mask{dim=filter_dim, dim2=5}
      mask prompts: dim "Filter Selection"; dim2 "Slice Selection"
  Weight Storage5 : Subsystem  mask{dim=filter_dim, dim2=6}
      mask prompts: dim "Filter Selection"; dim2 "Slice Selection"
  Weight Storage6 : Subsystem  mask{dim=filter_dim, dim2=7}
      mask prompts: dim "Filter Selection"; dim2 "Slice Selection"
  Weight Storage7 : Subsystem  mask{dim=filter_dim, dim2=8}
      mask prompts: dim "Filter Selection"; dim2 "Slice Selection"
  Weight Storage8 : Subsystem  mask{dim=filter_dim, dim2=9}
      mask prompts: dim "Filter Selection"; dim2 "Slice Selection"
  Weight Storage9 : Subsystem  mask{dim=filter_dim, dim2=10}
      mask prompts: dim "Filter Selection"; dim2 "Slice Selection"
  samplesOut : Outport
  validOut : Outport  Port=2
  wires:
  Data Type Conversion/1 -> samplesOut/1
  Demux/1 -> MAC0/2(samplesIn)
  MAC0/1(dataOut) -> Add/1
  Delay1/1 -> MAC14/3(validIn), MAC15/3(validIn), MAC13/3(validIn), MAC12/3(validIn), MAC11/3(validIn), MAC10/3(validIn), MAC9/3(validIn), MAC8/3(validIn), MAC7/3(validIn), MAC6/3(validIn), MAC5/3(validIn), MAC4/3(validIn), MAC3/3(validIn), MAC2/3(validIn), MAC1/3(validIn), MAC0/3(validIn)
  vectorIn/1 -> Delay/1
  Delay/1 -> Demux/1
  HDL Counter/1 -> Weight Storage 0/1(count_Weights), Weight Storage1/1(count_Weights), Weight Storage2/1(count_Weights), Weight Storage3/1(count_Weights), Weight Storage4/1(count_Weights), Weight Storage5/1(count_Weights), Weight Storage6/1(count_Weights), Weight Storage7/1(count_Weights), Weight Storage8/1(count_Weights), Weight Storage9/1(count_Weights), Weight Storage10/1(count_Weights), Weight Storage11/1(count_Weights), Weight Storage12/1(count_Weights), Weight Storage13/1(count_Weights), Weight Storage14/1(count_Weights), Weight Storage15/1(count_Weights)  "countWeights"
  validIn/1 -> Delay1/1, HDL Counter/1
  Weight Storage 0/1(weightsOut) -> MAC0/1(countWeights)
  Add/1 -> Data Type Conversion/1
  Weight Storage1/1(weightsOut) -> MAC1/1(countWeights)
  MAC1/1(dataOut) -> Add/2
  Demux/2 -> MAC1/2(samplesIn)
  Weight Storage2/1(weightsOut) -> MAC2/1(countWeights)
  MAC2/1(dataOut) -> Add/3
  Demux/3 -> MAC2/2(samplesIn)
  Weight Storage3/1(weightsOut) -> MAC3/1(countWeights)
  MAC3/1(dataOut) -> Add/4
  Demux/4 -> MAC3/2(samplesIn)
  Weight Storage4/1(weightsOut) -> MAC4/1(countWeights)
  MAC4/1(dataOut) -> Add/5
  Demux/5 -> MAC4/2(samplesIn)
  Weight Storage5/1(weightsOut) -> MAC5/1(countWeights)
  MAC5/1(dataOut) -> Add/6
  Demux/6 -> MAC5/2(samplesIn)
  Weight Storage6/1(weightsOut) -> MAC6/1(countWeights)
  MAC6/1(dataOut) -> Add/7
  Demux/7 -> MAC6/2(samplesIn)
  Weight Storage7/1(weightsOut) -> MAC7/1(countWeights)
  MAC7/1(dataOut) -> Add/8
  Demux/8 -> MAC7/2(samplesIn)
  Weight Storage8/1(weightsOut) -> MAC8/1(countWeights)
  MAC8/1(dataOut) -> Add/9
  Demux/9 -> MAC8/2(samplesIn)
  Weight Storage9/1(weightsOut) -> MAC9/1(countWeights)
  MAC9/1(dataOut) -> Add/10
  Demux/10 -> MAC9/2(samplesIn)
  Weight Storage10/1(weightsOut) -> MAC10/1(countWeights)
  MAC10/1(dataOut) -> Add/11
  Demux/11 -> MAC10/2(samplesIn)
  Weight Storage11/1(weightsOut) -> MAC11/1(countWeights)
  MAC11/1(dataOut) -> Add/12
  Demux/12 -> MAC11/2(samplesIn)
  Weight Storage12/1(weightsOut) -> MAC12/1(countWeights)
  MAC12/1(dataOut) -> Add/13
  Demux/13 -> MAC12/2(samplesIn)
  Weight Storage13/1(weightsOut) -> MAC13/1(countWeights)
  MAC13/1(dataOut) -> Add/14
  Demux/14 -> MAC13/2(samplesIn)
  Weight Storage14/1(weightsOut) -> MAC14/1(countWeights)
  MAC14/1(dataOut) -> Add/15
  Demux/15 -> MAC14/2(samplesIn)
  Weight Storage15/1(weightsOut) -> MAC15/1(countWeights)
  MAC15/1(dataOut) -> Add/16
  Demux/16 -> MAC15/2(samplesIn)
  MAC0/2(validOut) -> validOut/1

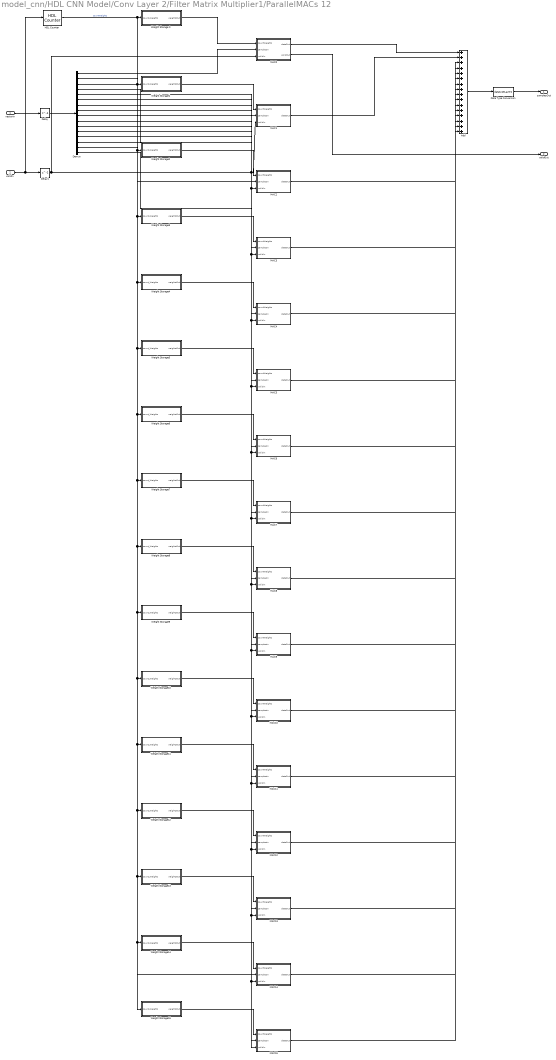
== system model_cnn/HDL CNN Model/Conv Layer 2/Filter Matrix Multiplier1/ParallelMACs 12 ==
  vectorIn : Inport
  validIn : Inport  Port=2
  Add : Sum  Inputs=++++++++++++++++  AccumDataTypeStr=accumoutdatatype2  OutDataTypeStr=accumoutdatatype2
  Data Type Conversion : DataTypeConversion  OutDataTypeStr=datatypeLayer2
  Delay : Delay  DelayLength=1
  Delay1 : Delay  DelayLength=1
  Demux : Demux  Outputs=16
  HDL Counter : hdlsllib/Sources/HDL Counter  CountType=Count limited  CountInit=0  CountStep=1  CountMax=24-1  CountFromType=Initial value  CountFrom=0  CountResetPort=off  CountLoadPort=off  CountEnbPort=on  CountDirPort=off  CountDataType=Unsigned  CountWordLen=ceil(log2(24))  CountFracLen=0  CountSampTime=1
  MAC0 : Subsystem
  MAC1 : Subsystem
  MAC10 : Subsystem
  MAC11 : Subsystem
  MAC12 : Subsystem
  MAC13 : Subsystem
  MAC14 : Subsystem
  MAC15 : Subsystem
  MAC2 : Subsystem
  MAC3 : Subsystem
  MAC4 : Subsystem
  MAC5 : Subsystem
  MAC6 : Subsystem
  MAC7 : Subsystem
  MAC8 : Subsystem
  MAC9 : Subsystem
  Weight Storage 0 : Subsystem  mask{dim=filter_dim, dim2=1}
      mask prompts: dim "Filter Selection"; dim2 "Slice Selection"
  Weight Storage1 : Subsystem  mask{dim=filter_dim, dim2=2}
      mask prompts: dim "Filter Selection"; dim2 "Slice Selection"
  Weight Storage10 : Subsystem  mask{dim=filter_dim, dim2=11}
      mask prompts: dim "Filter Selection"; dim2 "Slice Selection"
  Weight Storage11 : Subsystem  mask{dim=filter_dim, dim2=12}
      mask prompts: dim "Filter Selection"; dim2 "Slice Selection"
  Weight Storage12 : Subsystem  mask{dim=filter_dim, dim2=13}
      mask prompts: dim "Filter Selection"; dim2 "Slice Selection"
  Weight Storage13 : Subsystem  mask{dim=filter_dim, dim2=14}
      mask prompts: dim "Filter Selection"; dim2 "Slice Selection"
  Weight Storage14 : Subsystem  mask{dim=filter_dim, dim2=15}
      mask prompts: dim "Filter Selection"; dim2 "Slice Selection"
  Weight Storage15 : Subsystem  mask{dim=filter_dim, dim2=16}
      mask prompts: dim "Filter Selection"; dim2 "Slice Selection"
  Weight Storage2 : Subsystem  mask{dim=filter_dim, dim2=3}
      mask prompts: dim "Filter Selection"; dim2 "Slice Selection"
  Weight Storage3 : Subsystem  mask{dim=filter_dim, dim2=4}
      mask prompts: dim "Filter Selection"; dim2 "Slice Selection"
  Weight Storage4 : Subsystem  mask{dim=filter_dim, dim2=5}
      mask prompts: dim "Filter Selection"; dim2 "Slice Selection"
  Weight Storage5 : Subsystem  mask{dim=filter_dim, dim2=6}
      mask prompts: dim "Filter Selection"; dim2 "Slice Selection"
  Weight Storage6 : Subsystem  mask{dim=filter_dim, dim2=7}
      mask prompts: dim "Filter Selection"; dim2 "Slice Selection"
  Weight Storage7 : Subsystem  mask{dim=filter_dim, dim2=8}
      mask prompts: dim "Filter Selection"; dim2 "Slice Selection"
  Weight Storage8 : Subsystem  mask{dim=filter_dim, dim2=9}
      mask prompts: dim "Filter Selection"; dim2 "Slice Selection"
  Weight Storage9 : Subsystem  mask{dim=filter_dim, dim2=10}
      mask prompts: dim "Filter Selection"; dim2 "Slice Selection"
  samplesOut : Outport
  validOut : Outport  Port=2
  wires:
  MAC0/2(validOut) -> validOut/1
  Demux/16 -> MAC15/2(samplesIn)
  MAC15/1(dataOut) -> Add/16
  Weight Storage15/1(weightsOut) -> MAC15/1(countWeights)
  Demux/15 -> MAC14/2(samplesIn)
  MAC14/1(dataOut) -> Add/15
  Weight Storage14/1(weightsOut) -> MAC14/1(countWeights)
  Demux/14 -> MAC13/2(samplesIn)
  MAC13/1(dataOut) -> Add/14
  Weight Storage13/1(weightsOut) -> MAC13/1(countWeights)
  Demux/13 -> MAC12/2(samplesIn)
  MAC12/1(dataOut) -> Add/13
  Weight Storage12/1(weightsOut) -> MAC12/1(countWeights)
  Demux/12 -> MAC11/2(samplesIn)
  MAC11/1(dataOut) -> Add/12
  Weight Storage11/1(weightsOut) -> MAC11/1(countWeights)
  Demux/11 -> MAC10/2(samplesIn)
  MAC10/1(dataOut) -> Add/11
  Weight Storage10/1(weightsOut) -> MAC10/1(countWeights)
  Demux/10 -> MAC9/2(samplesIn)
  MAC9/1(dataOut) -> Add/10
  Weight Storage9/1(weightsOut) -> MAC9/1(countWeights)
  Demux/9 -> MAC8/2(samplesIn)
  MAC8/1(dataOut) -> Add/9
  Weight Storage8/1(weightsOut) -> MAC8/1(countWeights)
  Demux/8 -> MAC7/2(samplesIn)
  MAC7/1(dataOut) -> Add/8
  Weight Storage7/1(weightsOut) -> MAC7/1(countWeights)
  Demux/7 -> MAC6/2(samplesIn)
  MAC6/1(dataOut) -> Add/7
  Weight Storage6/1(weightsOut) -> MAC6/1(countWeights)
  Demux/6 -> MAC5/2(samplesIn)
  MAC5/1(dataOut) -> Add/6
  Weight Storage5/1(weightsOut) -> MAC5/1(countWeights)
  Demux/5 -> MAC4/2(samplesIn)
  MAC4/1(dataOut) -> Add/5
  Weight Storage4/1(weightsOut) -> MAC4/1(countWeights)
  Demux/4 -> MAC3/2(samplesIn)
  MAC3/1(dataOut) -> Add/4
  Weight Storage3/1(weightsOut) -> MAC3/1(countWeights)
  Demux/3 -> MAC2/2(samplesIn)
  MAC2/1(dataOut) -> Add/3
  Weight Storage2/1(weightsOut) -> MAC2/1(countWeights)
  Demux/2 -> MAC1/2(samplesIn)
  MAC1/1(dataOut) -> Add/2
  Weight Storage1/1(weightsOut) -> MAC1/1(countWeights)
  Add/1 -> Data Type Conversion/1
  Weight Storage 0/1(weightsOut) -> MAC0/1(countWeights)
  validIn/1 -> HDL Counter/1, Delay1/1
  HDL Counter/1 -> Weight Storage15/1(count_Weights), Weight Storage14/1(count_Weights), Weight Storage13/1(count_Weights), Weight Storage12/1(count_Weights), Weight Storage11/1(count_Weights), Weight Storage10/1(count_Weights), Weight Storage9/1(count_Weights), Weight Storage8/1(count_Weights), Weight Storage7/1(count_Weights), Weight Storage6/1(count_Weights), Weight Storage5/1(count_Weights), Weight Storage4/1(count_Weights), Weight Storage3/1(count_Weights), Weight Storage2/1(count_Weights), Weight Storage1/1(count_Weights), Weight Storage 0/1(count_Weights)  "countWeights"
  Delay/1 -> Demux/1
  vectorIn/1 -> Delay/1
  Delay1/1 -> MAC0/3(validIn), MAC1/3(validIn), MAC2/3(validIn), MAC3/3(validIn), MAC4/3(validIn), MAC5/3(validIn), MAC6/3(validIn), MAC7/3(validIn), MAC8/3(validIn), MAC9/3(validIn), MAC10/3(validIn), MAC11/3(validIn), MAC12/3(validIn), MAC13/3(validIn), MAC15/3(validIn), MAC14/3(validIn)
  MAC0/1(dataOut) -> Add/1
  Demux/1 -> MAC0/2(samplesIn)
  Data Type Conversion/1 -> samplesOut/1
